simulink model "sim_final"  (R2023b)
settings: Solver=FixedStepAuto  StartTime=0.0  StopTime=simtime  FixedStep=0.01  RelTol=1e-3
InitFcn:
  | if type == 1
  |     name = NEDC;
  | elseif type == 2
  |     name = CAFE;
  | elseif type == 3
  |     name = CNBUS;
  | elseif type == 4
  |     name = EUDC;
  | elseif type == 5
  |     name = FTP_75;
  | elseif type == 6
  |     name = HWFET;
  | elseif type == 7
  |     name = JC10;
  | elseif type == 8
  |     name = JC10_15;
  | elseif type == 9
  |     name = JC15;
  | elseif type == 10
  |     name = UDC;
  | end
  | tlen = size(name,1);
  | if simtimeflag
  |     simtime=tlen;
  | else
  |     fname = name;
  |     % i = ceil(basicsimtime/tlen);
  |     for i=1:ceil(basicsimtime/tlen)
  |         for j=1:tlen
  |             name(j+(i-1)*tlen,1)=fname(j,1)+(i-1)*tlen;
  |             name(j+(i-1)*tlen,2)=fname(j,2);
  |         end
  |     end
  |     simtime = basicsimtime;
  | end
undefined symbols (not defined in the file or in its folder): A, Cd, DiscIntNeverNeededParam, f, m, R_cha_SOC, R_dch_SOC, Vocv_cha_SOC
settings Model: Creator=ThinkPad  LastModifiedBy=ThinkPad

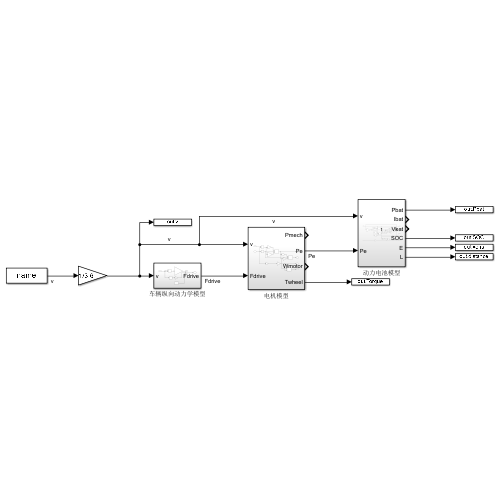
[thumbnail: Simulink's stored preview of the top-level diagram]
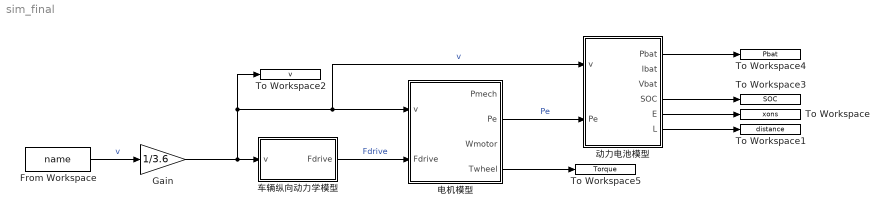
== system sim_final ==
  From Workspace : FromWorkspace  VariableName=name
  Gain : Gain  Gain=1/3.6
  To Workspace : ToWorkspace  VariableName=xons  SaveFormat=Timeseries  SampleTime=-1
  To Workspace1 : ToWorkspace  VariableName=distance  SaveFormat=Timeseries  SampleTime=-1
  To Workspace2 : ToWorkspace  VariableName=v  SaveFormat=Timeseries  SampleTime=-1
  To Workspace3 : ToWorkspace  VariableName=SOC  SaveFormat=Timeseries  SampleTime=-1
  To Workspace4 : ToWorkspace  VariableName=Pbat  SaveFormat=Timeseries  SampleTime=-1
  To Workspace5 : ToWorkspace  VariableName=Torque  SaveFormat=Timeseries  SampleTime=-1
  动力电池模型 : Subsystem
  电机模型 : Subsystem
  车辆纵向动力学模型 : Subsystem
  wires:
  From Workspace/1 -> Gain/1  "v"
  车辆纵向动力学模型/1(Fdrive) -> 电机模型/2(Fdrive)  "Fdrive"
  电机模型/2(Pe) -> 动力电池模型/2(Pe)  "Pe"
  动力电池模型/1(Pbat) -> To Workspace4/1
  动力电池模型/4(SOC) -> To Workspace3/1
  Gain/1 -> To Workspace2/1, 动力电池模型/1(v), 电机模型/1(v), 车辆纵向动力学模型/1(v)  "v"
  动力电池模型/5(E) -> To Workspace/1
  动力电池模型/6(L) -> To Workspace1/1
  电机模型/4(Twheel) -> To Workspace5/1

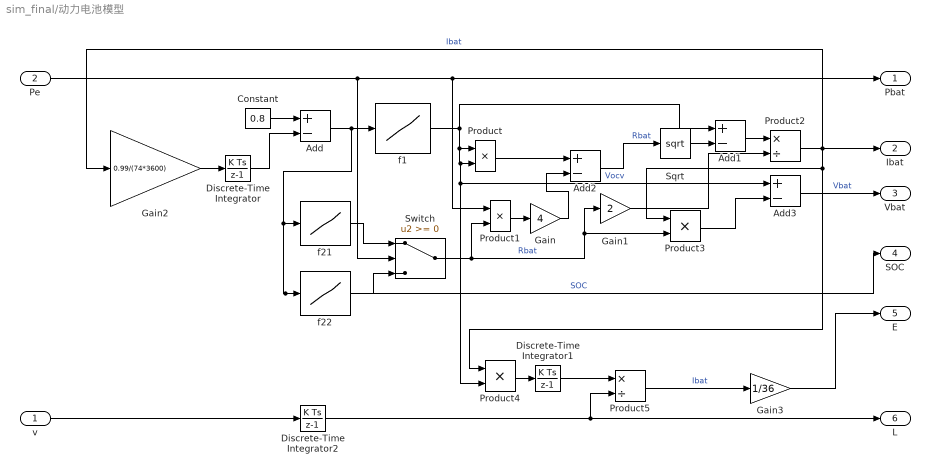
== system sim_final/动力电池模型 ==
  v : Inport
  Pe : Inport  Port=2
  Add{,1..3} (4 alike) : Sum  Inputs=+-
  Constant : Constant  Value=0.8
  Discrete-Time Integrator : DiscreteIntegrator  SampleTime=-1  ICPrevOutput=DiscIntNeverNeededParam  ICPrevScaledInput=DiscIntNeverNeededParam
  Discrete-Time Integrator1 : DiscreteIntegrator  SampleTime=-1  ICPrevOutput=DiscIntNeverNeededParam  ICPrevScaledInput=DiscIntNeverNeededParam
  Discrete-Time Integrator2 : DiscreteIntegrator  SampleTime=-1  ICPrevOutput=DiscIntNeverNeededParam  ICPrevScaledInput=DiscIntNeverNeededParam
  Gain : Gain  Gain=4
  Gain1 : Gain  Gain=2
  Gain2 : Gain  Gain=0.99/(74*3600)
  Gain3 : Gain  Gain=1/36
  Product{,1,3..4} (4 alike) : Product
  Product2 : Product  Inputs=*/
  Product5 : Product  Inputs=*/
  Sqrt : Sqrt
  Switch : Switch  SaturateOnIntegerOverflow=off  InputSameDT=off
  f1 : Lookup_n-D  NumberOfTableDimensions=1  BreakpointsForDimension1=Vocv_cha_SOC(:,1)  Table=Vocv_cha_SOC(:,2)  InternalRulePriority=Speed  RndMeth=Simplest
  f21 : Lookup_n-D  NumberOfTableDimensions=1  BreakpointsForDimension1=R_dch_SOC(:,1)  Table=R_dch_SOC(:,2)  InternalRulePriority=Speed  RndMeth=Simplest
  f22 : Lookup_n-D  NumberOfTableDimensions=1  BreakpointsForDimension1=R_cha_SOC(:,1)  Table=R_cha_SOC(:,2)  InternalRulePriority=Speed  RndMeth=Simplest
  Pbat : Outport
  Ibat : Outport  Port=2
  Vbat : Outport  Port=3
  SOC : Outport  Port=4
  E : Outport  Port=5
  L : Outport  Port=6
  wires:
  Product2/1 -> Product3/1, Product4/1, Ibat/1, Gain2/1  "Ibat"
  f1/1 -> Product/1, Add3/1, Product4/2, Product/2, Add1/1  "Vocv"
  Pe/1 -> Pbat/1, Product1/1, Switch/2
  v/1 -> Discrete-Time Integrator2/1
  Discrete-Time Integrator2/1 -> L/1, Product5/2
  Switch/1 -> Product3/2, Gain1/1, Product1/2  "Rbat"
  Add/1 -> f21/1, SOC/1, f22/1, f1/1  "SOC"
  Product/1 -> Add2/1
  Product3/1 -> Add3/2
  Product4/1 -> Discrete-Time Integrator1/1
  Gain2/1 -> Discrete-Time Integrator/1
  Add1/1 -> Product2/1
  Constant/1 -> Add/1
  Gain1/1 -> Product2/2
  f21/1 -> Switch/1
  Add3/1 -> Vbat/1  "Vbat"
  Product1/1 -> Gain/1
  f22/1 -> Switch/3
  Discrete-Time Integrator1/1 -> Product5/1
  Gain/1 -> Add2/2
  Discrete-Time Integrator/1 -> Add/2
  Sqrt/1 -> Add1/2
  Product5/1 -> Gain3/1  "Ibat"
  Gain3/1 -> E/1
  Add2/1 -> Sqrt/1  "Rbat"

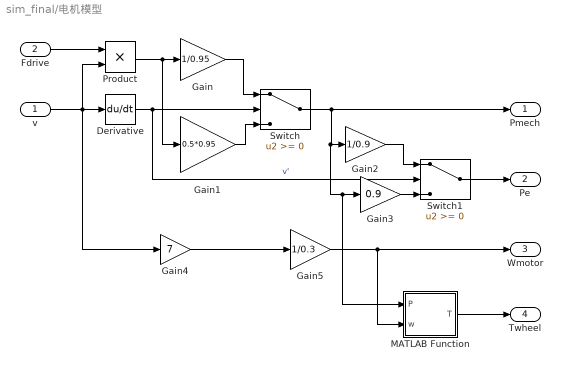
== system sim_final/电机模型 ==
  v : Inport
  Fdrive : Inport  Port=2
  Derivative : Derivative
  Gain : Gain  Gain=1/0.95
  Gain1 : Gain  Gain=0.5*0.95
  Gain2 : Gain  Gain=1/0.9
  Gain3 : Gain  Gain=0.9
  Gain4 : Gain  Gain=7
  Gain5 : Gain  Gain=1/0.3
  MATLAB Function : MATLAB Function  TreatAsAtomicUnit=on
  Product : Product
  Switch : Switch  SaturateOnIntegerOverflow=off  InputSameDT=off
  Switch1 : Switch  SaturateOnIntegerOverflow=off  InputSameDT=off
  Pmech : Outport
  Pe : Outport  Port=2
  Wmotor : Outport  Port=3
  Twheel : Outport  Port=4
  wires:
  Switch/1 -> Pmech/1, MATLAB Function/1(P), Gain3/1, Gain2/1
  Gain1/1 -> Switch/3
  Gain5/1 -> MATLAB Function/2(w), Wmotor/1
  Switch1/1 -> Pe/1
  Derivative/1 -> Switch1/2, Switch/2  "v'"
  Gain2/1 -> Switch1/1
  MATLAB Function/1(T) -> Twheel/1
  Gain/1 -> Switch/1
  Fdrive/1 -> Product/1
  v/1 -> Gain4/1, Product/2, Derivative/1
  Product/1 -> Gain1/1, Gain/1
  Gain4/1 -> Gain5/1
  Gain3/1 -> Switch1/3

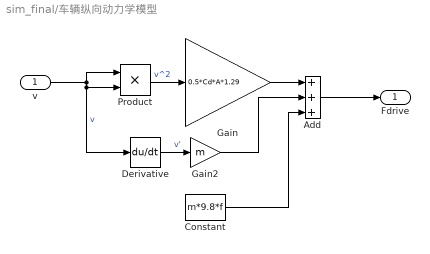
== system sim_final/车辆纵向动力学模型 ==
  v : Inport
  Add : Sum  Inputs=+++
  Constant : Constant  Value=m*9.8*f
  Derivative : Derivative
  Gain : Gain  Gain=0.5*Cd*A*1.29
  Gain2 : Gain  Gain=m
  Product : Product
  Fdrive : Outport
  wires:
  Gain/1 -> Add/1
  Derivative/1 -> Gain2/1  "v'"
  Constant/1 -> Add/3
  Add/1 -> Fdrive/1
  Gain2/1 -> Add/2
  v/1 -> Product/1, Product/2, Derivative/1  "v"
  Product/1 -> Gain/1  "v^2"

== matlab function sim_final/电机模型/MATLAB Function ==
  data: P input; w input; T output
function T = fcn(P,w)
if w
    T = P/w;
else
    T=0;
end
